simulink model "actual_model_v1"  (R2022a)
settings: Solver=ode23t  StartTime=0.0  StopTime=10  FixedStep=0.001  RelTol=1e-3
undefined symbols (not defined in the file or in its folder): A, A_hat, B, B_hat, C, C_lqe, C_lqr, Const_input, D, D_hat, Kr, x_des
settings Model: Creator=asmax  LastModifiedBy=asmax
settings SolverCC: EnableFixedStepZeroCrossing=on

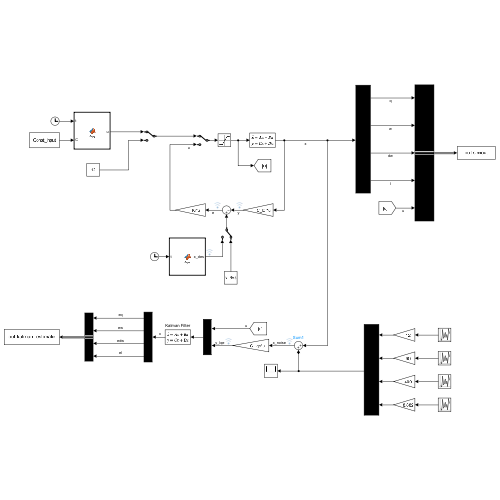
[thumbnail: Simulink's stored preview of the top-level diagram]
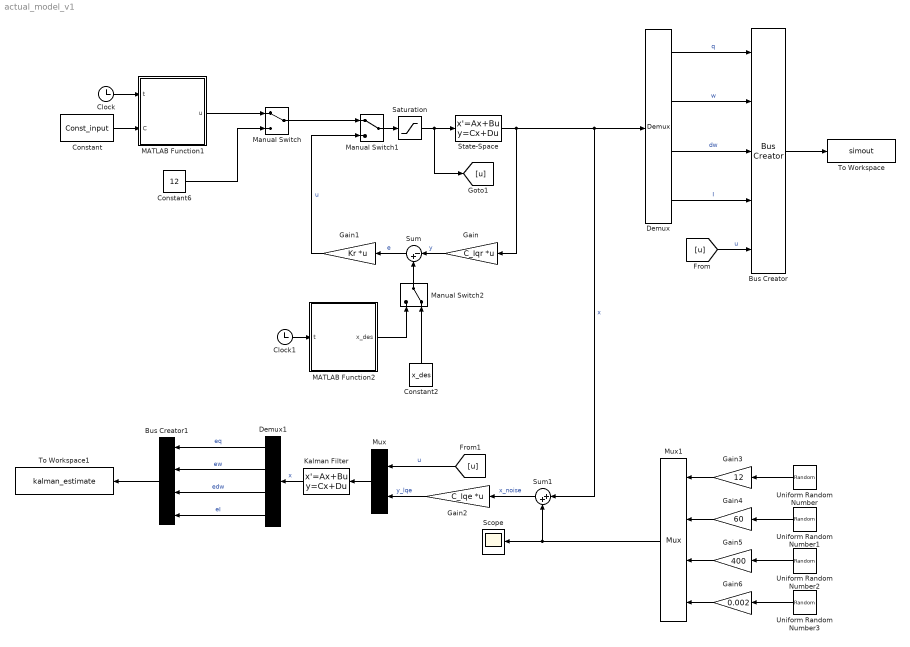
== system actual_model_v1 ==
  Bus Creator : BusCreator  Inputs=5
  Bus Creator1 : BusCreator  Inputs=4
  Clock : Clock
  Clock1 : Clock
  Constant : Constant  Value=Const_input
  Constant2 : Constant  Value=x_des
  Constant6 : Constant  Value=12
  Demux : Demux
  Demux1 : Demux
  Gain : Gain  Gain=C_lqr  Multiplication=Matrix(K*u)
  Gain1 : Gain  Gain=Kr  Multiplication=Matrix(K*u)
  Gain2 : Gain  Gain=C_lqe  Multiplication=Matrix(K*u)
  Gain3 : Gain  Gain=12
  Gain4 : Gain  Gain=60
  Gain5 : Gain  Gain=400
  Gain6 : Gain  Gain=0.002
  Kalman Filter : StateSpace  A=A_hat  B=B_hat  C=eye(4)  D=D_hat  InitialCondition=[0 0 0 0]'
  MATLAB Function1 : MATLAB Function  TreatAsAtomicUnit=on
  MATLAB Function2 : MATLAB Function  TreatAsAtomicUnit=on
  Manual Switch : ManualSwitch
  Manual Switch1 : ManualSwitch
  Manual Switch2 : ManualSwitch  CurrentSetting=0
  Mux : Mux  Inputs=2
  Mux1 : Mux
  Saturation : Saturate  UpperLimit=15  LowerLimit=-15
  Scope : Scope
  State-Space : StateSpace  A=A  B=B  C=C  D=D  InitialCondition=[0 0 0 0]'
  Sum : Sum  Inputs=|-+
  Sum1 : Sum  Inputs=|++
  To Workspace : ToWorkspace  VariableName=simout  SaveFormat=Timeseries  SampleTime=-1
  To Workspace1 : ToWorkspace  VariableName=kalman_estimate  SaveFormat=Timeseries  SampleTime=-1
  Uniform Random Number{,1..3} (4 alike) : UniformRandomNumber  SampleTime=0.01
  wires:
  Clock/1 -> MATLAB Function1/1(t)
  MATLAB Function1/1(u) -> Manual Switch/1
  Constant6/1 -> Manual Switch/2
  Constant/1 -> MATLAB Function1/2(C)
  State-Space/1 -> Gain/1, Sum1/1, Demux/1  "x"
  Bus Creator/1 -> To Workspace/1
  Demux/2 -> Bus Creator/2  "w"
  Demux/1 -> Bus Creator/1  "q"
  [u] -> Bus Creator/5  "u"
  Gain/1 -> Sum/1  "y"
  Manual Switch1/1 -> Saturation/1
  Gain1/1 -> Manual Switch1/2  "u"
  Manual Switch/1 -> Manual Switch1/1
  Sum/1 -> Gain1/1  "e"
  Demux/3 -> Bus Creator/3  "dw"
  Clock1/1 -> MATLAB Function2/1(t)
  Manual Switch2/1 -> Sum/2
  Constant2/1 -> Manual Switch2/2
  MATLAB Function2/1(x_des) -> Manual Switch2/1
  Saturation/1 -> [u], State-Space/1
  Demux/4 -> Bus Creator/4  "I"
  Mux/1 -> Kalman Filter/1
  [u] -> Mux/1  "u"
  Gain2/1 -> Mux/2  "y_lqe"
  Kalman Filter/1 -> Demux1/1  "x"
  Demux1/2 -> Bus Creator1/2  "ew"
  Demux1/1 -> Bus Creator1/1  "eq"
  Demux1/3 -> Bus Creator1/3  "edw"
  Demux1/4 -> Bus Creator1/4  "eI"
  Bus Creator1/1 -> To Workspace1/1
  Sum1/1 -> Gain2/1  "x_noise"
  Mux1/1 -> Sum1/2, Scope/1
  Uniform Random Number/1 -> Gain3/1
  Uniform Random Number1/1 -> Gain4/1
  Uniform Random Number2/1 -> Gain5/1
  Uniform Random Number3/1 -> Gain6/1
  Gain3/1 -> Mux1/1
  Gain4/1 -> Mux1/2
  Gain5/1 -> Mux1/3
  Gain6/1 -> Mux1/4

== matlab function actual_model_v1/MATLAB Function1 ==
  data: t input; u output; C input
function u = fcn(t, C)

% w = 4;
% A = 6;
% B = 6;
% fi = 3.1415;
% u = A * cos(w * t + fi) + B;

w = C(3);
A = C(1);
B = C(2);
fi = C(4);
u = A * cos(w * t + fi) + B;

== matlab function actual_model_v1/MATLAB Function2 ==
  data: t input; x_des output
function x_des = fcn(t)

w = 2;
A = 400;
B = A;
fi = 3.1415;
% w_des = A * cos(w * t + fi) + B;
w_des = -A*w * sin(w * t + fi);

w = 2;
A = 400;
B = A;
fi = 3.1415;
q_des = A * cos(w * t + fi) + B;

% x_des = [0 w_des 0 0]';
% x_des = [q_des 0 0 0]';
x_des = [q_des w_des 0 0]';
